simulink model "IW_Motor_0"  (R2023b)
settings: Solver=FixedStepAuto  StartTime=0.0  StopTime=inf  RelTol=1e-3  EnableMultiTasking=on
libraries: arduinomotorcarrierlib x1, eeGeneralControl x1, mkrmotorcarrierlib x1
settings Model: ExtModeTrigDuration=2  Creator=bkhusain
settings SolverCC: AlgebraicLoopSolver=TrustRegion
settings OptimizationCC: EnhancedBackFolding=on  PassReuseOutputArgsThreshold=0  MaxStackSize=64  OptimizeBlockOrder=speed  DifferentSizesBufferReuse=on  OptimizationCustomize=off
settings DebuggingCC: ParameterTunabilityLossMsg=error  UnconnectedInputMsg=warning  UnconnectedOutputMsg=warning  UnconnectedLineMsg=warning
settings HardwareCC: ProdBitPerPointer=32  ProdBitPerSizeT=32  ProdBitPerPtrDiffT=32  ProdLargestAtomicInteger=Long  ProdLargestAtomicFloat=Double  ProdWordSize=32  ProdHWDeviceType=ARM Compatible->ARM Cortex  UseEmbeddedCoderFeatures=off  UseSimulinkCoderFeatures=off
settings ModelReferenceCC: EnableRefExpFcnMdlSchedulingChecks=on
settings SFSimCC: MATLABDynamicMemAlloc=off
settings RTWCC: Description=Embedded Coder  SystemTargetFile=ert.tlc  HardwareBoard=Arduino Nano 33 IoT  TemplateMakefile=ert_default_tmf  Toolchain=Arduino ARM  BuildConfiguration=Faster Runs  DLArmComputeVersion=19.05
settings CodeAppCC: ForceParamTrailComments=on  OperatorAnnotations=on
settings ERTTargetCC: ERTCustomFileBanners=off  SupportContinuousTime=on  SupportNonInlinedSFcns=on  RemoveResetFunc=off  SupportVariableSizeSignals=on  ModelStepFunctionPrototypeControlCompliant=off  ExtModeStaticAllocSize=8192

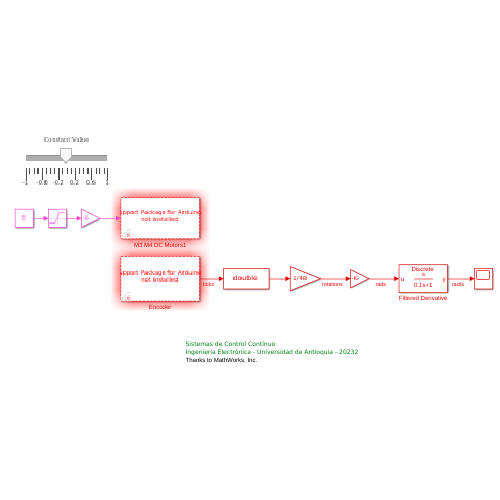
[thumbnail: Simulink's stored preview of the top-level diagram]
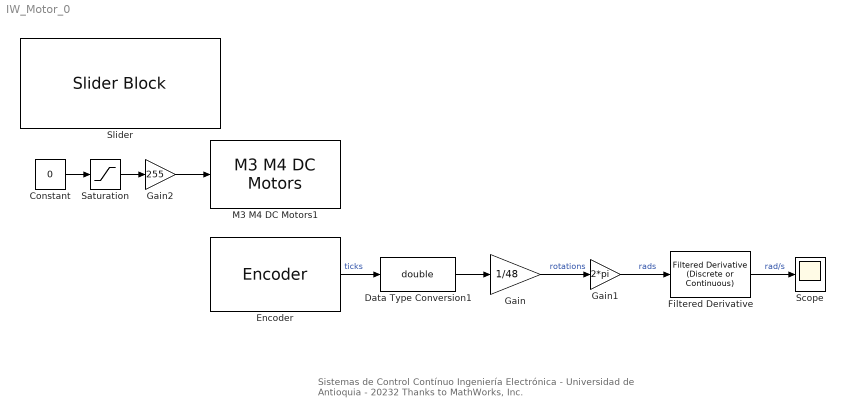
== system IW_Motor_0 ==
  note: Sistemas de Control Contínuo
      | Ingeniería Electrónica - Universidad de Antioquia - 20232
      | Thanks to MathWorks, Inc.
  Constant : Constant  Value=0  SampleTime=0.01
  Data Type Conversion1 : DataTypeConversion  OutDataTypeStr=double  SaturateOnIntegerOverflow=off  RndMeth=Floor
  Encoder : arduinomotorcarrierlib/Encoder  SlaveAddress=uint8( hex2dec( '66' ) )  blockPlatform=ARDUINO  Encoder=1  ShowSpeed=off  ResetOption=on  SampleTime=0.01
  "Filtered Derivative " : eeGeneralControl/Filtered Derivative (Discrete or Continuous)  K=1  T=0.1  B=inf  A=-inf  minRatio=10  init_option=Inherited from block input  x0=0  Ts=0.01
  Gain : Gain  Gain=1/48
  Gain1 : Gain  Gain=2*pi
  Gain2 : Gain  Gain=255
  M3 M4 DC Motors1 : mkrmotorcarrierlib/M3 M4 DC Motors  MotorNumber=M3  forwardPinNumber=3  reversePinNumber=2
  Saturation : Saturate  UpperLimit=1  LowerLimit=-1
  Scope : Scope
  Slider : SliderBlock  ScaleMin=-1  ScaleMax=1
  wires:
  "Filtered Derivative "/1 -> Scope/1  "rad/s"
  Gain/1 -> Gain1/1  "rotations"
  Gain1/1 -> "Filtered Derivative "/1  "rads"
  Encoder/1 -> Data Type Conversion1/1  "ticks"
  Data Type Conversion1/1 -> Gain/1
  Gain2/1 -> M3 M4 DC Motors1/1
  Constant/1 -> Saturation/1
  Saturation/1 -> Gain2/1
